simulink model "spiBitbang_complete_v2_2"  (R2013b)
settings: Solver=FixedStepDiscrete  StartTime=0.0  StopTime=5e-3  FixedStep=Ts  RelTol=1e-3
StopFcn:
  | run('spiBitBanging_process.m')
model workspace (MAT data in the model file):
  Ts = 1e-06
  periSam = 20
undefined symbols (not defined in the file or in its folder): High, rxdata
libraries: simulink_extras x17, dspswit3 x8, simulink x7, embdlinuxlib x4, dspsnks4 x3, dspsigops x1
settings Model: VariantConfigurationObject=RxSubsystem  Creator=mainster  LastModifiedBy=mainster
settings DataIOCC: SignalLogging=off  DSMLogging=off
settings DebuggingCC: UnderspecifiedInitializationDetection=Simplified
settings ConfigurationSet: Description=SimMechanics 2G

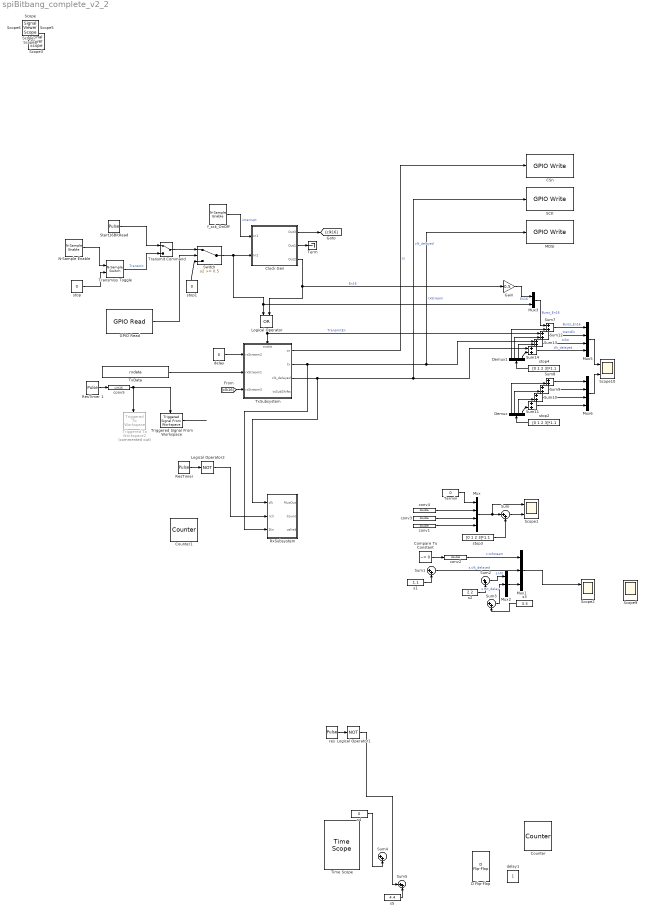
== system spiBitbang_complete_v2_2 ==
  CSn : embdlinuxlib/GPIO Write  board=Model B Rev2  gpio=8  direction=Output  blockPlatform=Raspberry Pi
  Clock Gen : Subsystem
  Compare To Constant : simulink/Logic and Bit Operations/Compare To Constant  relop=~=  const=0  OutDataTypeStr=boolean
  Counter : dspswit3/Counter  Direction=Up  CountEvent=Rising edge  CounterSize=User defined  MaxCount=20  InitialCount=0  Output=Count and Hit  HitValue=16  ResetInput=on  SamplesPerFrame=1  Ts=1  CntDtype=double  HitDtype=Logical
  Counter1 : dspswit3/Counter  Direction=Up  CountEvent=Rising edge  CounterSize=User defined  MaxCount=255  InitialCount=0  Output=Count and Hit  HitValue=[15 16 30 31 32]  ResetInput=on  SamplesPerFrame=1  Ts=1  CntDtype=double  HitDtype=Logical
  D Flip-Flop : simulink_extras/Flip Flops/D Flip-Flop
  Demux : Demux
  Demux1 : Demux
  GPIO Read : embdlinuxlib/GPIO Read  board=Model B Rev2  gpio=9  internalResistor=Off  sampleTime=0.1  direction=Input  blockPlatform=Raspberry Pi
  Gain : Gain  Gain=0.5  OutDataTypeStr=double
  Logical Operator : Logic  Operator=OR  AllPortsSameDT=off  OutDataTypeStr=boolean
  Logical Operator1 : Logic  Operator=NOT  IconShape=distinctive  AllPortsSameDT=off  OutDataTypeStr=boolean
  Logical Operator2 : Logic  Operator=NOT  IconShape=distinctive  AllPortsSameDT=off  OutDataTypeStr=boolean
  MOSI : embdlinuxlib/GPIO Write  board=Model B Rev2  gpio=10  direction=Output  blockPlatform=Raspberry Pi
  Mux : Mux
  Mux1 : Mux  Inputs=3
  Mux2 : Mux  Inputs=3
  Mux3 : Mux  Inputs=2
  Mux5 : Mux
  Mux6 : Mux
  N-Sample Enable : dspswit3/N-Sample Enable  N=70  ActiveLevel=High (1)  reset=off  TriggerType=Rising edge  Ts=-1  DataType=Logical
  "ResTimer " : DiscretePulseGenerator  Period=1200  PulseWidth=50  PhaseDelay=70  SampleTime=Ts
  ResTimer 1 : DiscretePulseGenerator  Period=100  PulseWidth=80  SampleTime=Ts
  RxSubsystem : Subsystem  VariantControl=Variant
  SCK : embdlinuxlib/GPIO Write  board=Model B Rev2  gpio=11  direction=Output  blockPlatform=Raspberry Pi
  Scope1 : Scope  NumInputPorts=2
      settings: ShowLegends=on  TimeRange=0.0015  YMin=-0.2~-0.2  YMax=5~15
  Scope10 : Scope  NumInputPorts=2
      settings: ShowLegends=on  YMin=-0.2~-0.2  YMax=5~15  SaveName=ScopeData3
  Scope2 : Scope  NumInputPorts=2
      settings: ShowLegends=on  TimeRange=0.0012  YMin=-0.2~-0.5  YMax=6.2~18  SaveName=ScopeData4
  Scope9 : Scope
      settings: TickLabels=on  ShowLegends=on  TimeRange=0.0012  YMin=0  YMax=23  SaveName=ScopeData2  SampleInput=on
  Start16BitRead : DiscretePulseGenerator  Period=500  PulseWidth=200  PhaseDelay=100  SampleTime=Ts
  Sum{,1..5} (6 alike) : Sum  Inputs=|++  LockScale=on
  Sum{7..14} (8 alike) : Sum  LockScale=on
  Switch : Switch  Threshold=0.5
  Term : Terminator
  Termin : Constant  Value=0  SampleTime=Ts
  Time Scope : TimeScope  NumInputPorts=4  DefaultConfigurationName=spbscopes.TimeScopeBlockCfg
      settings: CopyFcn=scopeextensions.ScopeBlock.onCoreBlockCopy(gcbh);  DeleteFcn=scopeextensions.ScopeBlock.callback(gcbh, 'onBlockDelete');  PreSaveFcn=scopeextensions.ScopeBlock.callback(gcbh, 'onModelSave');  NameChangeFcn=scopeextensions.ScopeBlock.callback(gcbh, 'onBlockRename');  DestroyFcn=scopeextensions.ScopeBlock.onBlockDestroy(gcbh)  CloseFcn=scopeextensions.ScopeBlock.callback(gcbh, 'onBlockClose');  PreDeleteFcn=scopeextensions.ScopeBlock.callback(gcbh, 'onBlockPreDelete');
  Transmiss Toggle : dspswit3/N-Sample Switch  N=300  reset=off  TriggerType=Rising edge  Ts=-1
  Transmit Command : ManualSwitch
  Triggered To Workspace2 : dspsnks4/Triggered To Workspace  Commented=on  TriggerType=Falling edge  VariableName=cap  Buffer=1000  Save2DMode=2-D array (concatenate along first dimension)
      settings: FixptAsFi=off
  Triggered Signal From Workspace : dspsigops/Triggered Signal From Workspace  Signal=rxdata  TriggerType=Falling edge  ic=0  SamplesPerFrame=1  OutputAfterFinalValue=Setting to zero
  TxData : Constant  Value=rxdata  OutDataTypeStr=uint16  SampleTime=Ts
  TxSubsystem : Subsystem  InitFcn=|
      | set_param('spiBitbang_complete_v2_2/TxSubsystem/cs/','InitialOutput','1')
      | set_param('spiBitbang_complete_v2_2/TxSubsystem/tx/','InitialOutput','0')
      | set_param('spiBitbang_complete_v2_2/TxSubsystem/txSubShifts','InitialOutput','0')
      | set_param('spiBitbang_complete_v2_2/TxSubsystem/clk_delayed','InitialOutput','0')
      settings: PropExecContextOutsideSubsystem=on
  conv{1..4} (4 alike) : DataTypeConversion  OutDataTypeStr=double  LockScale=on
  conv5 : DataTypeConversion  OutDataTypeStr=uint16  LockScale=on
  delay : Constant  Value=0  SampleTime=Ts
  delay1 : Constant  SampleTime=Ts
  f_sck_OnOff : dspswit3/N-Sample Enable  N=1  ActiveLevel=High (1)  reset=off  TriggerType=Falling edge  Ts=-1  DataType=Boolean
  res : DiscretePulseGenerator  Period=1000  PulseWidth=10  PhaseDelay=500  SampleTime=Ts
  s1 : Constant  Value=1.1  SampleTime=Ts
  s2 : Constant  Value=2.2  SampleTime=Ts
  s3 : Constant  Value=3.3  SampleTime=Ts
  s4 : Constant  Value=0  SampleTime=Ts
  s5 : Constant  Value=4.4  SampleTime=Ts
  stop : Constant  Value=0  OutDataTypeStr=Inherit: Inherit via back propagation  SampleTime=Ts
  stop1 : Constant  Value=0  OutDataTypeStr=Inherit: Inherit via back propagation  SampleTime=Ts
  stop2 : Constant  Value=[0 1 2 3]*1.1  SampleTime=Ts
  stop3 : Constant  Value=[0 1 2 3]*1.1  SampleTime=Ts
  stop4 : Constant  Value=[0 1 2 3]*1.1  SampleTime=Ts
  Scope : SignalViewerScope  IOType=viewer  NumInputPorts=3  RefreshTime=0.035000
      settings: ShowLegends=on  TimeRange=0.0005  YMin=-5~-5~-5  YMax=5~5~5
  Scope3 : SignalViewerScope  IOType=viewer  RefreshTime=0.035000
  Scope5 : SignalViewerScope  IOType=viewer  NumInputPorts=3  LegendLocations=|  RefreshTime=0.035000
      | 0.82061     0.88408     0.20293    0.077088
      | 0.87358     0.60048     0.13389     0.04354
      | 0.82864     0.29053     0.19247     0.04354
      settings: ShowLegends=on  TimeRange=0.0006  YMin=-5~-5~-5  YMax=5~5~5  SaveName=ScopeData2
  Scope6 : SignalViewerScope  IOType=viewer  RefreshTime=0.035000
      settings: SaveName=ScopeData3
  Scope7 : SignalViewerScope  IOType=viewer  LegendLocations="0.83596      0.7245     0.13305     0.16299"  RefreshTime=0.035000
      settings: ShowLegends=on  TimeRange=0.0011  YMin=-0.2  YMax=3.5  SaveName=ScopeData4
  Scope8 : SignalViewerScope  IOType=viewer  LegendLocations="0.85063     0.85718     0.13567    0.083065"  RefreshTime=0.035000
      settings: ShowLegends=on  SaveName=ScopeData5
  wires:
  f_sck_OnOff/1 -> Clock Gen/1(In1)  "interrupt"
  Sum/1 -> Scope1/2
  Mux/1 -> Scope1/1, Sum/1
  N-Sample Enable/1 -> Transmiss Toggle/1
  stop/1 -> Transmiss Toggle/2
  Transmiss Toggle/1 -> Transmit Command/2  "Transmit"
  Start16BitRead/1 -> Transmit Command/1
  Clock Gen/1(Out3) -> [clk16]
  delay/1 -> TxSubsystem/1(rxStream2)
  stop3/1 -> Sum/2
  conv1/1 -> Mux/4
  s1/1 -> Sum1/2
  Sum1/1 -> Mux1/2  "s.clk_delayed"
  conv3/1 -> Mux/3
  conv4/1 -> Mux/2
  Compare To Constant/1 -> conv2/1
  Mux1/1 -> Scope2/1
  conv2/1 -> Mux1/1  "c.txStream"
  res/1 -> Logical Operator1/1
  Clock Gen/2(Out1) -> Term/1
  Termin/1 -> Mux/1
  [clk16] -> TxSubsystem/3(rxStream3)
  s2/1 -> Sum2/2
  s3/1 -> Sum3/2
  Sum2/1 -> Mux2/1  "s.Hit"
  Mux2/1 -> Mux1/3
  Sum3/1 -> Mux2/2  "s.Hit_delay"
  s4/1 -> Sum4/2
  Logical Operator1/1 -> Sum5/1
  s5/1 -> Sum5/2
  Logical Operator/1 -> TxSubsystem/Enable, Sum12/1  "TransmitEn"
  Mux6/1 -> Scope10/2
  Sum8/1 -> Mux6/1
  Sum9/1 -> Mux6/2
  Sum10/1 -> Mux6/3
  Sum11/1 -> Mux6/4
  Demux/4 -> Sum11/2
  Demux/3 -> Sum10/2
  Demux/2 -> Sum9/2
  Demux/1 -> Sum8/2
  stop2/1 -> Demux/1
  Sum12/1 -> Mux5/2  "transEn"
  Sum13/1 -> Mux5/3  "txStr"
  Sum14/1 -> Mux5/4  "clk_delayed"
  Demux1/4 -> Sum14/2
  Demux1/3 -> Sum13/2
  Demux1/2 -> Sum12/2
  Demux1/1 -> Sum7/2
  stop4/1 -> Demux1/1
  Mux5/1 -> Scope10/1
  Transmit Command/1 -> Switch/1
  Switch/1 -> Logical Operator/1, Mux3/2, Clock Gen/2(In2)
  Clock Gen/3(Out2) -> Logical Operator/2, Gain/1  "En16"
  TxSubsystem/2(tx) -> MOSI/1, Sum13/1, RxSubsystem/3(Din)  "txStream"
  TxSubsystem/3(clk_delayed) -> RxSubsystem/1(clk), SCK/1, Sum14/1  "clk_delayed"
  Gain/1 -> Mux3/1  "En16"
  Sum7/1 -> Mux5/1  "Burst_En16"
  Mux3/1 -> Sum7/1  "Burst_En16"
  "ResTimer "/1 -> Logical Operator2/1
  Logical Operator2/1 -> RxSubsystem/2(!clr)
  ? -> Triggered To Workspace2/1
  ResTimer 1/1 -> conv5/1
  Triggered Signal From Workspace/1 -> ?
  conv5/1 -> Triggered Signal From Workspace/Trigger, Triggered To Workspace2/Trigger
  TxData/1 -> TxSubsystem/2(rxStream1)
  TxSubsystem/1(cs) -> CSn/1  "cs"
  GPIO Read/1 -> Switch/2
  stop1/1 -> Switch/3

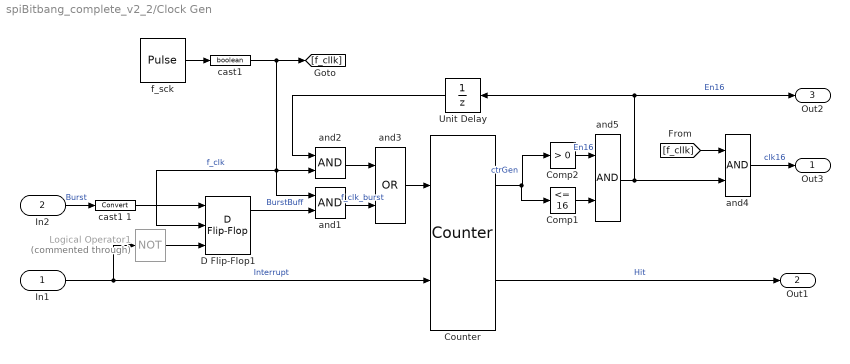
== system spiBitbang_complete_v2_2/Clock Gen ==
  In1 : Inport
  In2 : Inport  Port=2
  Comp1 : simulink/Logic and Bit Operations/Compare To Constant  relop=<=  const=16  OutDataTypeStr=boolean
  Comp2 : simulink/Logic and Bit Operations/Compare To Constant  relop=>  const=0  OutDataTypeStr=boolean
  Counter : dspswit3/Counter  Direction=Up  CountEvent=Rising edge  CounterSize=User defined  MaxCount=16  InitialCount=0  Output=Count and Hit  HitValue=periSam/4  ResetInput=on  SamplesPerFrame=1  Ts=1  CntDtype=double  HitDtype=Logical
  D Flip-Flop1 : simulink_extras/Flip Flops/D Flip-Flop
  Logical Operator1 : Logic  Commented=through  Operator=NOT  IconShape=distinctive  AllPortsSameDT=off  OutDataTypeStr=boolean
  Unit Delay : UnitDelay  SampleTime=-1
  and{1..2,4..5} (4 alike) : Logic  AllPortsSameDT=off  OutDataTypeStr=boolean
      settings: AttributesFormatString=%<Tag>
  and3 : Logic  Operator=OR  AllPortsSameDT=off  OutDataTypeStr=boolean
      settings: AttributesFormatString=%<Tag>
  "cast1 " : DataTypeConversion  OutDataTypeStr=boolean
  cast1 1 : DataTypeConversion
  f_sck : DiscretePulseGenerator  Period=periSam  PulseWidth=periSam/2  SampleTime=Ts
      settings: AttributesFormatString=|
      | Period =%<Period>
      | sTime=%<SampleTime>
      | Delay=%<PhaseDelay>
  Out3 : Outport
  Out1 : Outport  Port=2
  Out2 : Outport  Port=3
  wires:
  "cast1 "/1 -> and1/1, D Flip-Flop1/2, and2/2, [f_cllk]  "f_clk"
  f_sck/1 -> "cast1 "/1
  In1/1 -> Logical Operator1/1, Counter/2  "Interrupt"
  and3/1 -> Counter/1
  and4/1 -> Out3/1  "clk16"
  and1/1 -> and3/2  "f_clk_burst"
  and2/1 -> and3/1
  Unit Delay/1 -> and2/1
  Counter/2 -> Out1/1  "Hit"
  [f_cllk] -> and4/1
  Counter/1 -> Comp1/1, Comp2/1  "ctrGen"
  and5/1 -> Unit Delay/1, Out2/1, and4/2  "En16"
  Comp2/1 -> and5/1  "En16"
  Comp1/1 -> and5/2
  cast1 1/1 -> D Flip-Flop1/1
  Logical Operator1/1 -> D Flip-Flop1/3
  In2/1 -> cast1 1/1  "Burst"
  D Flip-Flop1/1 -> and1/2  "BurstBuff"

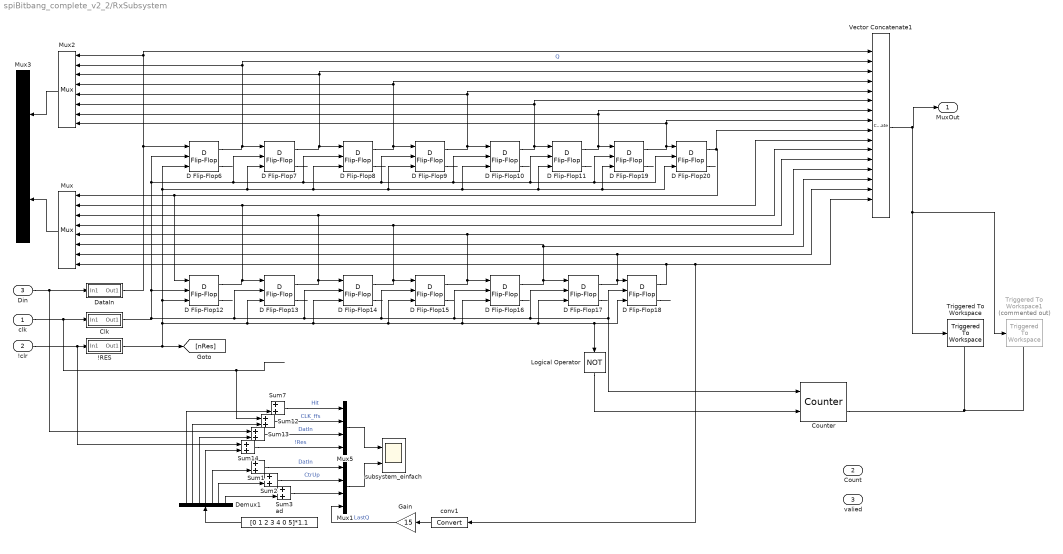
== system spiBitbang_complete_v2_2/RxSubsystem ==
  clk : Inport
  !clr : Inport  Port=2
  Din : Inport  Port=3
  !RES : Subsystem
  Clk : Subsystem
  Counter : dspswit3/Counter  Direction=Up  CountEvent=Rising edge  CounterSize=User defined  MaxCount=255  InitialCount=0  Output=Count and Hit  HitValue=[15 16 30 31 32]  ResetInput=on  SamplesPerFrame=1  Ts=1  CntDtype=double  HitDtype=Logical
  D Flip-Flop{6..20} (15 alike) : simulink_extras/Flip Flops/D Flip-Flop
  DataIn : Subsystem
  Demux1 : Demux  Outputs=7
  Gain : Gain  Gain=15
  Logical Operator : Logic  Operator=NOT  IconShape=distinctive  AllPortsSameDT=off  OutDataTypeStr=boolean
  Mux : Mux  Inputs=8
  Mux1 : Mux
  Mux2 : Mux  Inputs=8
  Mux3 : Mux  Inputs=2
  Mux5 : Mux
  Sum{1..3,7,12..14} (7 alike) : Sum  LockScale=on
  Triggered To Workspace : dspsnks4/Triggered To Workspace  TriggerType=Rising edge  VariableName=RxDataRaw  Buffer=1000  Save2DMode=2-D array (concatenate along first dimension)
      settings: FixptAsFi=off
  Triggered To Workspace1 : dspsnks4/Triggered To Workspace  Commented=on  TriggerType=Falling edge  VariableName=RxDataRaw2  Buffer=1000  Save2DMode=2-D array (concatenate along first dimension)
      settings: FixptAsFi=off
  Vector Concatenate1 : Concatenate  NumInputs=16
  ad : Constant  Value=[0 1 2 3 4 0 5]*1.1  SampleTime=Ts
  conv1 : DataTypeConversion
  subsystem_einfach : Scope  NumInputPorts=2
      settings: ShowLegends=on  YMin=-0.2~-1  YMax=5~20  SaveName=ScopeData7
  MuxOut : Outport
  Count : Outport  Port=2
  valied : Outport  Port=3
  wires:
  Gain/1 -> Mux1/4  "LastQ"
  conv1/1 -> Gain/1
  Mux1/1 -> subsystem_einfach/2
  Sum3/1 -> Mux1/3
  Sum2/1 -> Mux1/2  "CtrUp"
  Sum1/1 -> Mux1/1  "DatIn"
  Demux1/7 -> Sum3/2
  Demux1/6 -> Sum2/2
  Demux1/5 -> Sum1/2
  Sum7/1 -> Mux5/1  "Hit"
  Mux5/1 -> subsystem_einfach/1
  ad/1 -> Demux1/1
  Demux1/1 -> Sum7/2
  Demux1/2 -> Sum12/2
  Demux1/3 -> Sum13/2
  Demux1/4 -> Sum14/2
  Sum14/1 -> Mux5/4  "!Res"
  Sum13/1 -> Mux5/3  "DatIn"
  Sum12/1 -> Mux5/2  "CLK_ffs"
  Clk/1(Out1) -> D Flip-Flop14/2, D Flip-Flop15/2, D Flip-Flop18/2, Counter/1, D Flip-Flop17/2, D Flip-Flop16/2, D Flip-Flop13/2, D Flip-Flop12/2, D Flip-Flop7/2, D Flip-Flop8/2, D Flip-Flop9/2, D Flip-Flop10/2, D Flip-Flop11/2, D Flip-Flop19/2, D Flip-Flop20/2, D Flip-Flop6/2
  DataIn/1(Out1) -> Vector Concatenate1/1, Mux2/1, D Flip-Flop6/1
  D Flip-Flop10/2 -> ?
  D Flip-Flop12/2 -> ?
  D Flip-Flop16/2 -> ?
  D Flip-Flop7/2 -> ?
  D Flip-Flop9/2 -> ?
  D Flip-Flop8/2 -> ?
  D Flip-Flop11/2 -> ?
  D Flip-Flop6/2 -> ?
  D Flip-Flop13/2 -> ?
  D Flip-Flop17/2 -> ?
  D Flip-Flop20/2 -> ?
  D Flip-Flop19/2 -> ?
  D Flip-Flop18/2 -> ?
  D Flip-Flop14/2 -> ?
  D Flip-Flop15/2 -> ?
  D Flip-Flop19/1 -> D Flip-Flop20/1, Vector Concatenate1/8, Mux2/8
  Mux2/1 -> Mux3/1
  D Flip-Flop20/1 -> Mux/1, D Flip-Flop12/1, Vector Concatenate1/9
  D Flip-Flop12/1 -> D Flip-Flop13/1, Vector Concatenate1/10, Mux/2
  Mux/1 -> Mux3/2
  D Flip-Flop15/1 -> D Flip-Flop16/1, Mux/5, Vector Concatenate1/13
  D Flip-Flop9/1 -> D Flip-Flop10/1, Vector Concatenate1/5, Mux2/5
  D Flip-Flop6/1 -> D Flip-Flop7/1, Mux2/2, Vector Concatenate1/2  "Q"
  D Flip-Flop18/1 -> Mux/8, Vector Concatenate1/16, conv1/1
  D Flip-Flop14/1 -> D Flip-Flop15/1, Mux/4, Vector Concatenate1/12
  D Flip-Flop10/1 -> D Flip-Flop11/1, Vector Concatenate1/6, Mux2/6
  D Flip-Flop8/1 -> D Flip-Flop9/1, Mux2/4, Vector Concatenate1/4
  D Flip-Flop11/1 -> D Flip-Flop19/1, Mux2/7, Vector Concatenate1/7
  D Flip-Flop17/1 -> D Flip-Flop18/1, Mux/7, Vector Concatenate1/15
  D Flip-Flop16/1 -> D Flip-Flop17/1, Mux/6, Vector Concatenate1/14
  D Flip-Flop13/1 -> D Flip-Flop14/1, Vector Concatenate1/11, Mux/3
  D Flip-Flop7/1 -> D Flip-Flop8/1, Vector Concatenate1/3, Mux2/3
  Vector Concatenate1/1 -> Triggered To Workspace/1, Triggered To Workspace1/1, MuxOut/1
  clk/1 -> Sum12/1, Clk/1(In1)
  Din/1 -> Sum13/1, DataIn/1(In1)
  !clr/1 -> Sum14/1, !RES/1(In1)
  !RES/1(Out1) -> [nRes], D Flip-Flop13/3, D Flip-Flop14/3, D Flip-Flop15/3, D Flip-Flop16/3, D Flip-Flop17/3, Logical Operator/1, D Flip-Flop18/3, D Flip-Flop12/3, D Flip-Flop7/3, D Flip-Flop8/3, D Flip-Flop9/3, D Flip-Flop10/3, D Flip-Flop11/3, D Flip-Flop20/3, D Flip-Flop19/3, D Flip-Flop6/3
  Logical Operator/1 -> Counter/2
  Counter/2 -> Triggered To Workspace1/Trigger, Triggered To Workspace/Trigger

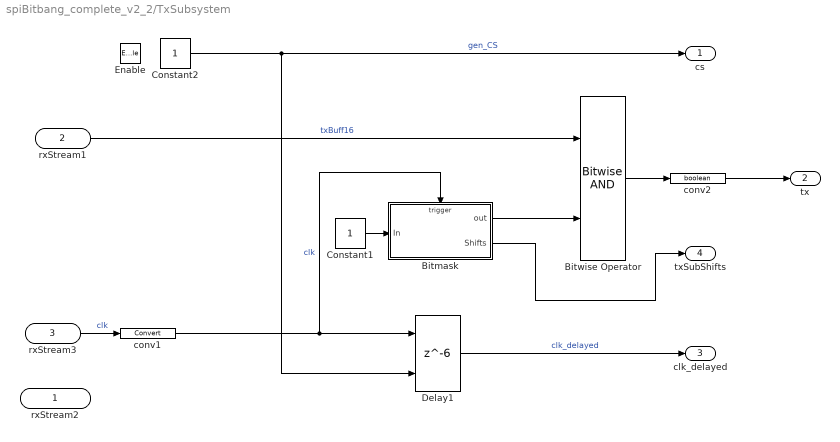
== system spiBitbang_complete_v2_2/TxSubsystem ==
  rxStream2 : Inport
  rxStream1 : Inport  Port=2  OutDataTypeStr=uint16
  rxStream3 : Inport  Port=3
  Enable : EnablePort  StatesWhenEnabling=reset
  Bitmask : Subsystem  TreatAsAtomicUnit=on
  Bitwise Operator : simulink/Logic and Bit Operations/Bitwise Operator  logicop=AND  UseBitMask=off  NumInputPorts=2  BitMask=bin2dec('11011001')  BitMaskRealWorld=Stored Integer
  Constant1 : Constant
  Constant2 : Constant
  Delay1 : Delay  DelayLength=6  InitialCondition=0  ExternalReset=Rising  InputProcessing=Inherited
      settings: InputPortMap=u0,r5
  conv1 : DataTypeConversion
  conv2 : DataTypeConversion  OutDataTypeStr=boolean
  cs : Outport  OutputWhenDisabled=reset  InitialOutput=1
  tx : Outport  Port=2  OutDataTypeStr=boolean  OutputWhenDisabled=reset  InitialOutput=0  LockScale=on
  clk_delayed : Outport  Port=3  OutputWhenDisabled=reset  InitialOutput=0
  txSubShifts : Outport  Port=4  OutputWhenDisabled=reset  InitialOutput=0
  wires:
  Constant2/1 -> cs/1, Delay1/2  "gen_CS"
  rxStream1/1 -> Bitwise Operator/1  "txBuff16"
  rxStream3/1 -> conv1/1  "clk"
  conv1/1 -> Bitmask/Trigger, Delay1/1  "clk"
  Constant1/1 -> Bitmask/1(In)
  Bitmask/1(out) -> Bitwise Operator/2
  Bitwise Operator/1 -> conv2/1
  Bitmask/2(Shifts) -> txSubShifts/1
  Delay1/1 -> clk_delayed/1  "clk_delayed"
  conv2/1 -> tx/1

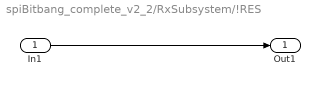
== system spiBitbang_complete_v2_2/RxSubsystem/!RES ==
  In1 : Inport
  Out1 : Outport
  wires:
  In1/1 -> Out1/1

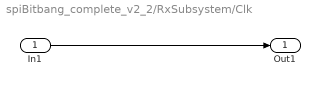
== system spiBitbang_complete_v2_2/RxSubsystem/Clk ==
  In1 : Inport
  Out1 : Outport
  wires:
  In1/1 -> Out1/1

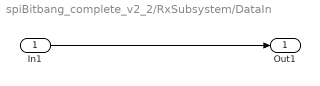
== system spiBitbang_complete_v2_2/RxSubsystem/DataIn ==
  In1 : Inport
  Out1 : Outport
  wires:
  In1/1 -> Out1/1

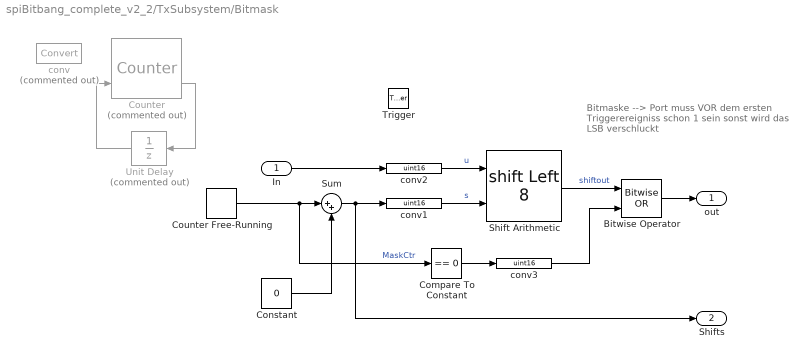
== system spiBitbang_complete_v2_2/TxSubsystem/Bitmask ==
  note: Bitmaske --> Port muss VOR dem ersten
      | Triggerereigniss schon 1 sein sonst wird
      | das LSB verschluckt
  In : Inport
  Trigger : TriggerPort  PortDimensions=1
  Bitwise Operator : simulink/Logic and Bit Operations/Bitwise Operator  logicop=OR  UseBitMask=off  NumInputPorts=2  BitMask=2  BitMaskRealWorld=Stored Integer
  Compare To Constant : simulink/Logic and Bit Operations/Compare To Constant  relop===  const=0  OutDataTypeStr=uint8
  Constant : Constant  Value=0  SampleTime=-1
  Counter : dspswit3/Counter  Commented=on  Direction=Up  CountEvent=Rising edge  CounterSize=User defined  MaxCount=16  InitialCount=1  Output=Count and Hit  HitValue=16  ResetInput=on  SamplesPerFrame=1  Ts=1  CntDtype=double  HitDtype=Logical
  Counter Free-Running : simulink/Sources/Counter Free-Running  NumBits=14  tsamp=-1
  Shift Arithmetic : ArithShift  BitShiftNumberSource=Input port  BitShiftNumber=8  BitShiftDirection=Left  DiagnosticForOORShift=Error
      settings: InputPortMap=u0,p1
  Sum : Sum  Inputs=|++
  Unit Delay : UnitDelay  Commented=on  SampleTime=-1
  conv : DataTypeConversion  Commented=on
  conv1 : DataTypeConversion  OutDataTypeStr=uint16
  conv2 : DataTypeConversion  OutDataTypeStr=uint16
  conv3 : DataTypeConversion  OutDataTypeStr=uint16
  out : Outport  InitialOutput=[1]
  Shifts : Outport  Port=2
  wires:
  Shift Arithmetic/1 -> Bitwise Operator/1  "shiftout"
  In/1 -> conv2/1
  Sum/1 -> Shifts/1, conv1/1
  Constant/1 -> Sum/2
  conv1/1 -> Shift Arithmetic/2  "s"
  conv2/1 -> Shift Arithmetic/1  "u"
  Counter/2 -> Unit Delay/1
  Unit Delay/1 -> Counter/2
  Counter Free-Running/1 -> Compare To Constant/1, Sum/1  "MaskCtr"
  Bitwise Operator/1 -> out/1
  Compare To Constant/1 -> conv3/1
  conv3/1 -> Bitwise Operator/2
